simulink model "matlab_exoskeleton"  (R2019b)
settings: Solver=VariableStepAuto  StartTime=0.0  StopTime=10.0  RelTol=1e-3
undefined symbols (not defined in the file): CAN_Device, PEAK, Serial_Port, Standard_Devices, System
libraries: sldrtlib x7, canmsglib x5
settings Model: Creator=wumin  LastModifiedBy=wumin

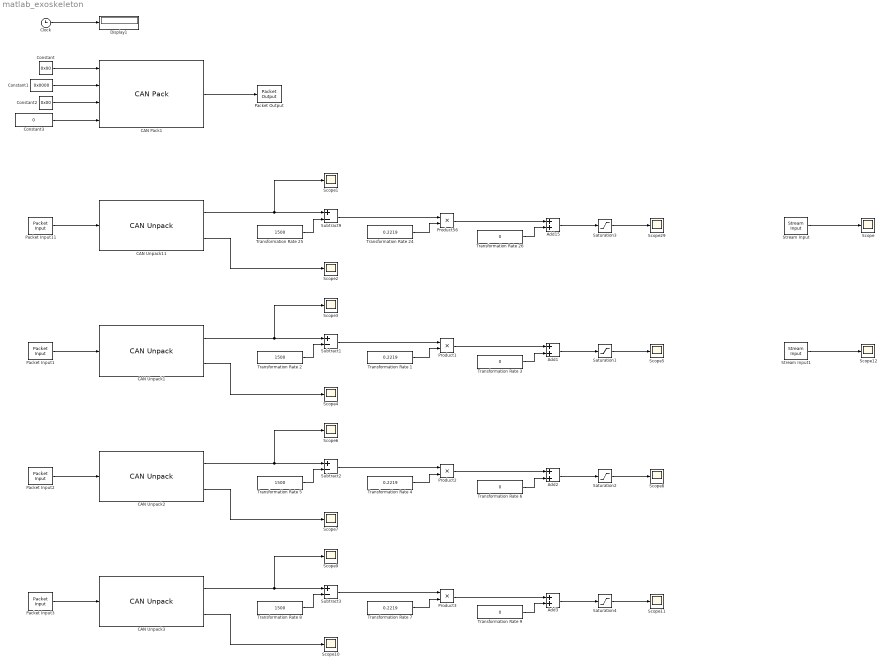
== system matlab_exoskeleton ==
  Add{1..3,15} (4 alike) : Sum
  CAN Pack1 : canmsglib/CAN Pack  MsgList=(none)  MsgName=CANopen Msg  MsgIDType=Standard (11-bit identifier)  MsgIdentifier=0x80  MsgLength=8  Remote=off  ApplyMinMax=off  BusOutput=off  SignalInfo={ 'Operation', '0', '8', 'LE', 'unsigned', 'Standard', '0', '1', '0', '-Inf', 'Inf'; 'Index', '8', '16', 'LE', 'unsigned', 'Standard', '0', '1', '0', '-Inf', 'Inf'; 'SubIndex', '24', '8', 'LE', 'unsigned', 'Standard', '0', '1', '0', '-Inf', 'Inf'; 'Data', '32', '32', 'LE', 'unsigned', 'Standard', '0', '1', '0', '-Inf', 'Inf' }
      settings: SourceProductName=Vehicle Network Toolbox  SourceProductBaseCode=VN  DataFormat=manually specified signals
  CAN Unpack{1..3,11} (4 alike) : canmsglib/CAN Unpack  MsgList=(none)  MsgName=CANopen Msg  MsgIDType=Standard (11-bit identifier)  MsgIdentifier=0x181  MsgLength=8  SignalInfo={ 'Sensor Raw Data', '0', '32', 'LE', 'unsigned', 'Standard', '0', '1', '0', '-Inf', 'Inf'; 'Sensor Calibrate Data', '32', '32', 'LE', 'unsigned', 'Standard', '0', '1', '0', '-Inf', 'Inf' }  IDPort=off  TimestampPort=off  ErrorPort=off  RemotePort=off  LengthPort=off  StatusPort=off  ApplyMinMax=off
      settings: SourceProductName=Vehicle Network Toolbox  SourceProductBaseCode=VN
  Clock : Clock
  Constant : Constant  Value=0x00  OutDataTypeStr=uint8  SampleTime=0
  Constant1 : Constant  Value=0x0000  OutDataTypeStr=uint16
  Constant2 : Constant  Value=0x00  OutDataTypeStr=uint8
  Constant3 : Constant  Value=0  OutDataTypeStr=uint32
  Display1 : Display
  Packet Input{1..3,11} (4 alike) : sldrtlib/Packet Input  SampleTime=0.001  MaxMissedTicks=10  ShowMissedTicks=off  YieldWhenWaiting=off  DrvName=PEAK-System/CAN_Device  DrvAddress=81  DrvOptions=[0 0 0 0 1000]  PacketSize=8  DataTypes='CAN_MESSAGE'  ShowReady=off  ShowError=off  PacketID=2048e0 + (double(0x181))  ByteOrder=1  ShowTimestamp=off
      settings: AttributesFormatString=PEAK-System\nCAN Device [81]  SourceProductName=Simulink Desktop Real-Time
  Packet Output : sldrtlib/Packet Output  SampleTime=-1  MaxMissedTicks=10  ShowMissedTicks=off  YieldWhenWaiting=off  DrvName=PEAK-System/CAN_Device  DrvAddress=81  DrvOptions=[0 0 0 0 1000]  PacketSize=8  DataTypes='CAN_MESSAGE'  ShowReady=off  ShowError=off  PacketID=2048e0 + (double(0x80))  ByteOrder=1  InitialValue=[]  FinalValue=[]
      settings: AttributesFormatString=PEAK-System\nCAN Device [81]  SourceProductName=Simulink Desktop Real-Time
  Product{1..3,56} (4 alike) : Product
  Saturation{1..4} (4 alike) : Saturate  UpperLimit=200  LowerLimit=-200
  Scope{,1..12,29} (14 alike) : Scope
  Stream Input : sldrtlib/Stream Input  SampleTime=0.001  MaxMissedTicks=10  ShowMissedTicks=off  YieldWhenWaiting=off  DrvName=Standard_Devices/Serial_Port  DrvAddress=1  DrvOptions=[115200 8 0 0 0 0 0 0]  DataTypes='double'  FormatString='%f'  Terminator={'\n'}  ShowReady=off  ShowError=off
      settings: AttributesFormatString=Serial Port [1]  SourceProductName=Simulink Desktop Real-Time  SourceProductBaseCode=WT
  Stream Input1 : sldrtlib/Stream Input  SampleTime=0.001  MaxMissedTicks=10  ShowMissedTicks=off  YieldWhenWaiting=off  DrvName=Standard_Devices/Serial_Port  DrvAddress=1  DrvOptions=[115200 8 0 0 0 0 0 0]  DataTypes='double'  FormatString='%f'  Terminator={'\n'}  ShowReady=off  ShowError=off
      settings: AttributesFormatString=Serial Port [1]  SourceProductName=Simulink Desktop Real-Time  SourceProductBaseCode=WT
  Subtract{1..3,9} (4 alike) : Sum  Inputs=+-
  Transformation Rate {1,4,7,24} (4 alike) : Constant  Value=0.2219
  Transformation Rate {2,5,8,25} (4 alike) : Constant  Value=1500
  Transformation Rate {3,6,9,26} (4 alike) : Constant  Value=0
  wires:
  CAN Pack1/1 -> Packet Output/1
  CAN Unpack11/2 -> Scope2/1
  Constant3/1 -> CAN Pack1/4
  Transformation Rate 26/1 -> Add15/2
  Constant2/1 -> CAN Pack1/3
  Constant/1 -> CAN Pack1/1
  Constant1/1 -> CAN Pack1/2
  Transformation Rate 24/1 -> Product56/2
  Packet Input11/1 -> CAN Unpack11/1
  CAN Unpack11/1 -> Scope1/1, Subtract9/1
  Transformation Rate 25/1 -> Subtract9/2
  Saturation3/1 -> Scope29/1
  Product56/1 -> Add15/1
  Add15/1 -> Saturation3/1
  Subtract9/1 -> Product56/1
  Clock/1 -> Display1/1
  Add1/1 -> Saturation1/1
  Subtract1/1 -> Product1/1
  Saturation1/1 -> Scope5/1
  Transformation Rate 2/1 -> Subtract1/2
  CAN Unpack1/1 -> Scope3/1, Subtract1/1
  Product1/1 -> Add1/1
  Transformation Rate 3/1 -> Add1/2
  CAN Unpack1/2 -> Scope4/1
  Transformation Rate 1/1 -> Product1/2
  Packet Input1/1 -> CAN Unpack1/1
  Add2/1 -> Saturation2/1
  Subtract2/1 -> Product2/1
  Saturation2/1 -> Scope8/1
  Transformation Rate 5/1 -> Subtract2/2
  CAN Unpack2/1 -> Scope6/1, Subtract2/1
  Product2/1 -> Add2/1
  Transformation Rate 6/1 -> Add2/2
  CAN Unpack2/2 -> Scope7/1
  Transformation Rate 4/1 -> Product2/2
  Packet Input2/1 -> CAN Unpack2/1
  Add3/1 -> Saturation4/1
  Subtract3/1 -> Product3/1
  Saturation4/1 -> Scope11/1
  Transformation Rate 8/1 -> Subtract3/2
  CAN Unpack3/1 -> Scope9/1, Subtract3/1
  Product3/1 -> Add3/1
  Transformation Rate 9/1 -> Add3/2
  CAN Unpack3/2 -> Scope10/1
  Transformation Rate 7/1 -> Product3/2
  Packet Input3/1 -> CAN Unpack3/1
  Stream Input/1 -> Scope/1
  Stream Input1/1 -> Scope12/1
